simulink model "AMPC_sCon"  (R2019b)
settings: Solver=FixedStepAuto  StartTime=0.0  StopTime=Time(end)  FixedStep=0.025  RelTol=1e-3
libraries: neural x47, mpclib x1, cstblocks x1
(part 2 of 2)

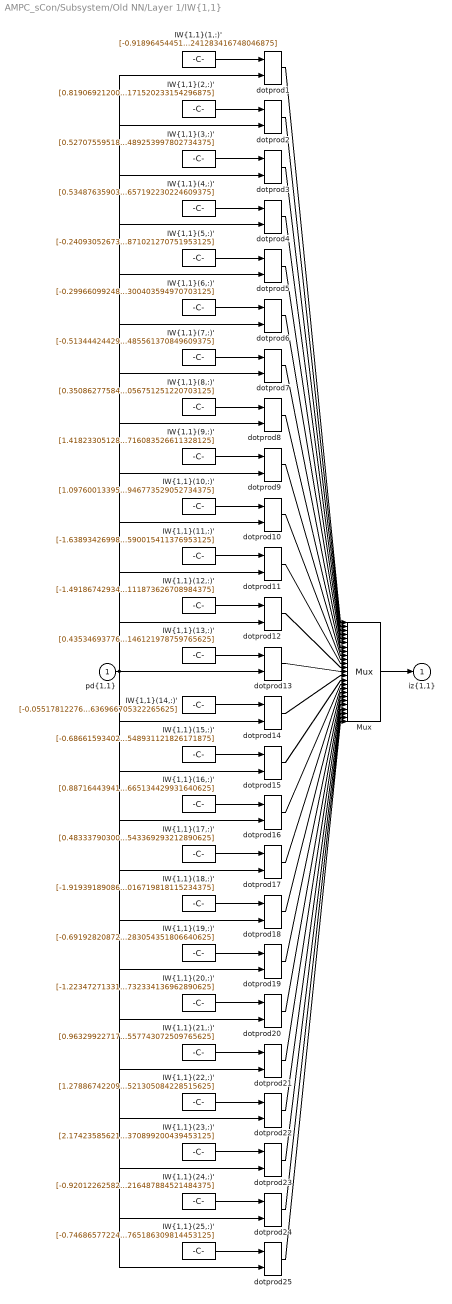
== system AMPC_sCon/Subsystem/Old NN/Layer 1/IW{1,1} ==
  "pd{1,1}" : Inport  PortDimensions=6
      mask Display: e = 0.06;c1 = [120 230 180]/255;c2 = ([120 230 180]+0)/(256+128);c3 = ([120 230 180]+128)/(256+128);patch([0 1 1 0],[0 0 1 1],c1);patch([0 1 1 1-e 1-e 0+e],[0 0 1 1-e 0+e 0+e],c2);patch([0 0 1 1-e 0+e 0+e],[0 1 1 1-e 1-e 0+e],c3);plot([0 1 1 0 0],[0 0 1 1 0]);
  "IW{1,1}(1,:)'" : Constant  Value=[-0.91896454451869669100005921791307628154754638671875;2.807406064374065923772150199511088430881500244140625;-0.32650530029088009609239406927372328937053680419921875;-0.68212399974366133559300351407728157937526702880859375;0.55443567787012237868538022667053155601024627685546875;-0.328157572076140435779478821132215671241283416748046875]
      mask Display: e = 0.06;c1 = [120 150 230]/255;c2 = ([120 150 230]+0)/383;c3 = ([120 150 230]+128)/383;patch([0 1 1 0],[0 0 1 1],c1);patch([0 1 1 1-e 1-e 0+e],[0 0 1 1-e 0+e 0+e],c2);patch([0 0 1 1-e 0+e 0+e],[0 1 1 1-e 1-e 0+e],c3);plot([0 1 1 0 0],[0 0 1 1 0]);disp('Weights');
  "IW{1,1}(10,:)'" : Constant  Value=[1.097600133959441226494391230517067015171051025390625;-0.07827061444567622039425458524419809691607952117919921875;-0.38990454765808413295502532491809688508510589599609375;0.46998928551050112023546034833998419344425201416015625;0.4354289920842753236485123125021345913410186767578125;-0.59819487501920798333543416447355411946773529052734375]
      mask Display: e = 0.06;c1 = [120 150 230]/255;c2 = ([120 150 230]+0)/383;c3 = ([120 150 230]+128)/383;patch([0 1 1 0],[0 0 1 1],c1);patch([0 1 1 1-e 1-e 0+e],[0 0 1 1-e 0+e 0+e],c2);patch([0 0 1 1-e 0+e 0+e],[0 1 1 1-e 1-e 0+e],c3);plot([0 1 1 0 0],[0 0 1 1 0]);disp('Weights');
  "IW{1,1}(11,:)'" : Constant  Value=[-1.6389342699858098217902124815736897289752960205078125;-0.7309100789032456635396783894975669682025909423828125;0.0018010659112654837758771275701974445837549865245819091796875;0.83129641458116487751084378032828681170940399169921875;-0.93893409236719238553092736765393055975437164306640625;0.084419703238978460735353337440756149590015411376953125]
      mask Display: e = 0.06;c1 = [120 150 230]/255;c2 = ([120 150 230]+0)/383;c3 = ([120 150 230]+128)/383;patch([0 1 1 0],[0 0 1 1],c1);patch([0 1 1 1-e 1-e 0+e],[0 0 1 1-e 0+e 0+e],c2);patch([0 0 1 1-e 0+e 0+e],[0 1 1 1-e 1-e 0+e],c3);plot([0 1 1 0 0],[0 0 1 1 0]);disp('Weights');
  "IW{1,1}(12,:)'" : Constant  Value=[-1.4918674293447633516507266904227435588836669921875;0.52049473620865904788246325551881454885005950927734375;-0.272842583889991330270419211956323124468326568603515625;-0.5921939615822207070294780351105146110057830810546875;-1.6000734146301442972770701089757494628429412841796875;-0.7163345210483613723084772573201917111873626708984375]
      mask Display: e = 0.06;c1 = [120 150 230]/255;c2 = ([120 150 230]+0)/383;c3 = ([120 150 230]+128)/383;patch([0 1 1 0],[0 0 1 1],c1);patch([0 1 1 1-e 1-e 0+e],[0 0 1 1-e 0+e 0+e],c2);patch([0 0 1 1-e 0+e 0+e],[0 1 1 1-e 1-e 0+e],c3);plot([0 1 1 0 0],[0 0 1 1 0]);disp('Weights');
  "IW{1,1}(13,:)'" : Constant  Value=[0.4353469377680905250116438764962367713451385498046875;-0.84085297783017975969954704851261340081691741943359375;-0.3262431999570882812378158632782287895679473876953125;-0.03343748267568195930987684505453216843307018280029296875;0.7569219535729778680632762188906781375408172607421875;-0.336770011411867520312313217800692655146121978759765625]
      mask Display: e = 0.06;c1 = [120 150 230]/255;c2 = ([120 150 230]+0)/383;c3 = ([120 150 230]+128)/383;patch([0 1 1 0],[0 0 1 1],c1);patch([0 1 1 1-e 1-e 0+e],[0 0 1 1-e 0+e 0+e],c2);patch([0 0 1 1-e 0+e 0+e],[0 1 1 1-e 1-e 0+e],c3);plot([0 1 1 0 0],[0 0 1 1 0]);disp('Weights');
  "IW{1,1}(14,:)'" : Constant  Value=[-0.055178122760997337648003480126135400496423244476318359375;-1.4381626335296340268854464738979004323482513427734375;0.1875648565884424356919879528504679910838603973388671875;-0.53640519002087516664545319144963286817073822021484375;-1.0068525371299339443709186525666154921054840087890625;0.160847593541183275789308027015067636966705322265625]
      mask Display: e = 0.06;c1 = [120 150 230]/255;c2 = ([120 150 230]+0)/383;c3 = ([120 150 230]+128)/383;patch([0 1 1 0],[0 0 1 1],c1);patch([0 1 1 1-e 1-e 0+e],[0 0 1 1-e 0+e 0+e],c2);patch([0 0 1 1-e 0+e 0+e],[0 1 1 1-e 1-e 0+e],c3);plot([0 1 1 0 0],[0 0 1 1 0]);disp('Weights');
  "IW{1,1}(15,:)'" : Constant  Value=[-0.686615934023023566368237879942171275615692138671875;0.426894044409089457037254078386467881500720977783203125;-0.60810228251544184985277752275578677654266357421875;0.1522748062778661870542151746121817268431186676025390625;-2.1099858845401460172297447570599615573883056640625;0.1713882654697056195924886878856341354548931121826171875]
      mask Display: e = 0.06;c1 = [120 150 230]/255;c2 = ([120 150 230]+0)/383;c3 = ([120 150 230]+128)/383;patch([0 1 1 0],[0 0 1 1],c1);patch([0 1 1 1-e 1-e 0+e],[0 0 1 1-e 0+e 0+e],c2);patch([0 0 1 1-e 0+e 0+e],[0 1 1 1-e 1-e 0+e],c3);plot([0 1 1 0 0],[0 0 1 1 0]);disp('Weights');
  "IW{1,1}(16,:)'" : Constant  Value=[0.88716443941147471452524086998892016708850860595703125;0.40313159970102241391742836640332825481891632080078125;-0.015657524645655340744809791431180201470851898193359375;-0.478263451738349443242981351431808434426784515380859375;0.3859891211729997717583273697528056800365447998046875;0.6315189817233604063773100278922356665134429931640625]
      mask Display: e = 0.06;c1 = [120 150 230]/255;c2 = ([120 150 230]+0)/383;c3 = ([120 150 230]+128)/383;patch([0 1 1 0],[0 0 1 1],c1);patch([0 1 1 1-e 1-e 0+e],[0 0 1 1-e 0+e 0+e],c2);patch([0 0 1 1-e 0+e 0+e],[0 1 1 1-e 1-e 0+e],c3);plot([0 1 1 0 0],[0 0 1 1 0]);disp('Weights');
  "IW{1,1}(17,:)'" : Constant  Value=[0.48333790300379242399486656722729094326496124267578125;0.0251588125096972210770207567520628799684345722198486328125;-0.67153040371300332100901187004637904465198516845703125;0.46244925298389250034603037420311011373996734619140625;-0.126361383991284270678079337812960147857666015625;-0.9536652713805617853637386360787786543369293212890625]
      mask Display: e = 0.06;c1 = [120 150 230]/255;c2 = ([120 150 230]+0)/383;c3 = ([120 150 230]+128)/383;patch([0 1 1 0],[0 0 1 1],c1);patch([0 1 1 1-e 1-e 0+e],[0 0 1 1-e 0+e 0+e],c2);patch([0 0 1 1-e 0+e 0+e],[0 1 1 1-e 1-e 0+e],c3);plot([0 1 1 0 0],[0 0 1 1 0]);disp('Weights');
  "IW{1,1}(18,:)'" : Constant  Value=[-1.919391890863494598562510873307473957538604736328125;2.760761832853932506992578055360354483127593994140625;0.166517652488541612054717688806704245507717132568359375;0.554430338119628718374087839038111269474029541015625;0.9634316882260487435729601202183403074741363525390625;-1.5238850536123587087189434896572493016719818115234375]
      mask Display: e = 0.06;c1 = [120 150 230]/255;c2 = ([120 150 230]+0)/383;c3 = ([120 150 230]+128)/383;patch([0 1 1 0],[0 0 1 1],c1);patch([0 1 1 1-e 1-e 0+e],[0 0 1 1-e 0+e 0+e],c2);patch([0 0 1 1-e 0+e 0+e],[0 1 1 1-e 1-e 0+e],c3);plot([0 1 1 0 0],[0 0 1 1 0]);disp('Weights');
  "IW{1,1}(19,:)'" : Constant  Value=[-0.69192820872236715512570981445605866611003875732421875;-1.0115896887588913255484612818690948188304901123046875;0.2082050329143752265270705947841634042561054229736328125;1.4276170938064451920723740840912796556949615478515625;0.60289644057316038594507290326873771846294403076171875;0.491245567452074427539088219418772496283054351806640625]
      mask Display: e = 0.06;c1 = [120 150 230]/255;c2 = ([120 150 230]+0)/383;c3 = ([120 150 230]+128)/383;patch([0 1 1 0],[0 0 1 1],c1);patch([0 1 1 1-e 1-e 0+e],[0 0 1 1-e 0+e 0+e],c2);patch([0 0 1 1-e 0+e 0+e],[0 1 1 1-e 1-e 0+e],c3);plot([0 1 1 0 0],[0 0 1 1 0]);disp('Weights');
  "IW{1,1}(2,:)'" : Constant  Value=[0.819069212007324409796638065017759799957275390625;1.4205841344905445478019601068808697164058685302734375;-0.2087539526108411480631588119649677537381649017333984375;0.5615055630163883204630792533862404525279998779296875;0.7621159660466625407337915021344088017940521240234375;-0.25482421381122211112568720636772923171520233154296875]
      mask Display: e = 0.06;c1 = [120 150 230]/255;c2 = ([120 150 230]+0)/383;c3 = ([120 150 230]+128)/383;patch([0 1 1 0],[0 0 1 1],c1);patch([0 1 1 1-e 1-e 0+e],[0 0 1 1-e 0+e 0+e],c2);patch([0 0 1 1-e 0+e 0+e],[0 1 1 1-e 1-e 0+e],c3);plot([0 1 1 0 0],[0 0 1 1 0]);disp('Weights');
  "IW{1,1}(20,:)'" : Constant  Value=[-1.223472713315403748168819220154546201229095458984375;1.02781452349469848428498153225518763065338134765625;-0.5016143513805861875454183973488397896289825439453125;-0.76512208370276379998387028535944409668445587158203125;-0.343872743653884926917640996180125512182712554931640625;-0.8302771328935032446594277644180692732334136962890625]
      mask Display: e = 0.06;c1 = [120 150 230]/255;c2 = ([120 150 230]+0)/383;c3 = ([120 150 230]+128)/383;patch([0 1 1 0],[0 0 1 1],c1);patch([0 1 1 1-e 1-e 0+e],[0 0 1 1-e 0+e 0+e],c2);patch([0 0 1 1-e 0+e 0+e],[0 1 1 1-e 1-e 0+e],c3);plot([0 1 1 0 0],[0 0 1 1 0]);disp('Weights');
  "IW{1,1}(21,:)'" : Constant  Value=[0.96329922717340188409451684492523781955242156982421875;-0.6551169661280218381449458320275880396366119384765625;-0.50582440032005393515390778702567331492900848388671875;0.046064824593341609226815336342042428441345691680908203125;1.406097969527585700433292004163376986980438232421875;-1.30481552967731406766915824846364557743072509765625]
      mask Display: e = 0.06;c1 = [120 150 230]/255;c2 = ([120 150 230]+0)/383;c3 = ([120 150 230]+128)/383;patch([0 1 1 0],[0 0 1 1],c1);patch([0 1 1 1-e 1-e 0+e],[0 0 1 1-e 0+e 0+e],c2);patch([0 0 1 1-e 0+e 0+e],[0 1 1 1-e 1-e 0+e],c3);plot([0 1 1 0 0],[0 0 1 1 0]);disp('Weights');
  "IW{1,1}(22,:)'" : Constant  Value=[1.2788674220914140189364616162492893636226654052734375;-0.499205108866402846867771359029575251042842864990234375;0.12542267272189933091652846997021697461605072021484375;-0.54779174719712830921025670249946415424346923828125;0.97010399881503683872097099083475768566131591796875;0.613862465609015917067381451488472521305084228515625]
      mask Display: e = 0.06;c1 = [120 150 230]/255;c2 = ([120 150 230]+0)/383;c3 = ([120 150 230]+128)/383;patch([0 1 1 0],[0 0 1 1],c1);patch([0 1 1 1-e 1-e 0+e],[0 0 1 1-e 0+e 0+e],c2);patch([0 0 1 1-e 0+e 0+e],[0 1 1 1-e 1-e 0+e],c3);plot([0 1 1 0 0],[0 0 1 1 0]);disp('Weights');
  "IW{1,1}(23,:)'" : Constant  Value=[2.1742358562138814903619277174584567546844482421875;0.7779663865511003972841308495844714343547821044921875;0.11376764528600201431540739349657087586820125579833984375;-0.321381834602109339726894177147187292575836181640625;0.31338586648281763213930162237375043332576751708984375;0.8184780163425291465983946181950159370899200439453125]
      mask Display: e = 0.06;c1 = [120 150 230]/255;c2 = ([120 150 230]+0)/383;c3 = ([120 150 230]+128)/383;patch([0 1 1 0],[0 0 1 1],c1);patch([0 1 1 1-e 1-e 0+e],[0 0 1 1-e 0+e 0+e],c2);patch([0 0 1 1-e 0+e 0+e],[0 1 1 1-e 1-e 0+e],c3);plot([0 1 1 0 0],[0 0 1 1 0]);disp('Weights');
  "IW{1,1}(24,:)'" : Constant  Value=[-0.920122625825073203742476835031993687152862548828125;1.7985903786357282374552823966951109468936920166015625;-0.449335796921472019338494874318712390959262847900390625;0.37211945524182443723049118489143438637256622314453125;-0.268179811625878616876406113078701309859752655029296875;-0.99187628535014782382717157815932296216487884521484375]
      mask Display: e = 0.06;c1 = [120 150 230]/255;c2 = ([120 150 230]+0)/383;c3 = ([120 150 230]+128)/383;patch([0 1 1 0],[0 0 1 1],c1);patch([0 1 1 1-e 1-e 0+e],[0 0 1 1-e 0+e 0+e],c2);patch([0 0 1 1-e 0+e 0+e],[0 1 1 1-e 1-e 0+e],c3);plot([0 1 1 0 0],[0 0 1 1 0]);disp('Weights');
  "IW{1,1}(25,:)'" : Constant  Value=[-0.7468657722437128665404770799796096980571746826171875;0.9514243031970905928318416044930927455425262451171875;-0.19912347847005718026736076353699900209903717041015625;0.42273079982580286095839028348564170300960540771484375;-0.454298439023558542348979472080827690660953521728515625;0.1158651407635991337219394381463644094765186309814453125]
      mask Display: e = 0.06;c1 = [120 150 230]/255;c2 = ([120 150 230]+0)/383;c3 = ([120 150 230]+128)/383;patch([0 1 1 0],[0 0 1 1],c1);patch([0 1 1 1-e 1-e 0+e],[0 0 1 1-e 0+e 0+e],c2);patch([0 0 1 1-e 0+e 0+e],[0 1 1 1-e 1-e 0+e],c3);plot([0 1 1 0 0],[0 0 1 1 0]);disp('Weights');
  "IW{1,1}(3,:)'" : Constant  Value=[0.52707559518076940729969237509067170321941375732421875;-1.35807461272378393601911739096976816654205322265625;0.6803855694700444711742193248937837779521942138671875;0.5457109471856937954470367913017980754375457763671875;-0.87266721000643909800231767803779803216457366943359375;0.354606028999767397547060454598977230489253997802734375]
      mask Display: e = 0.06;c1 = [120 150 230]/255;c2 = ([120 150 230]+0)/383;c3 = ([120 150 230]+128)/383;patch([0 1 1 0],[0 0 1 1],c1);patch([0 1 1 1-e 1-e 0+e],[0 0 1 1-e 0+e 0+e],c2);patch([0 0 1 1-e 0+e 0+e],[0 1 1 1-e 1-e 0+e],c3);plot([0 1 1 0 0],[0 0 1 1 0]);disp('Weights');
  "IW{1,1}(4,:)'" : Constant  Value=[0.5348763590344882690175154493772424757480621337890625;-2.94460120006832237748994884896092116832733154296875;0.25881394439468252688385518922586925327777862548828125;-0.988869737367270573713540215976536273956298828125;-1.34291304141692702245336477062664926052093505859375;0.8873294643855762497963723944849334657192230224609375]
      mask Display: e = 0.06;c1 = [120 150 230]/255;c2 = ([120 150 230]+0)/383;c3 = ([120 150 230]+128)/383;patch([0 1 1 0],[0 0 1 1],c1);patch([0 1 1 1-e 1-e 0+e],[0 0 1 1-e 0+e 0+e],c2);patch([0 0 1 1-e 0+e 0+e],[0 1 1 1-e 1-e 0+e],c3);plot([0 1 1 0 0],[0 0 1 1 0]);disp('Weights');
  "IW{1,1}(5,:)'" : Constant  Value=[-0.2409305267371661951614214558503590524196624755859375;1.3517602448933578873635497075156308710575103759765625;0.671714233157041373800666406168602406978607177734375;0.1699364545961201400370299552378128282725811004638671875;1.4733154643789483362326109272544272243976593017578125;0.44108263254802881903060551849193871021270751953125]
      mask Display: e = 0.06;c1 = [120 150 230]/255;c2 = ([120 150 230]+0)/383;c3 = ([120 150 230]+128)/383;patch([0 1 1 0],[0 0 1 1],c1);patch([0 1 1 1-e 1-e 0+e],[0 0 1 1-e 0+e 0+e],c2);patch([0 0 1 1-e 0+e 0+e],[0 1 1 1-e 1-e 0+e],c3);plot([0 1 1 0 0],[0 0 1 1 0]);disp('Weights');
  "IW{1,1}(6,:)'" : Constant  Value=[-0.29966099248417654710152646657661534845829010009765625;2.155080979873955637771132387570105493068695068359375;-0.5456468341177356240478957261075265705585479736328125;1.29078953244448957349277407047338783740997314453125;0.66091237151677351135958815575577318668365478515625;0.7268233797996483946946000287425704300403594970703125]
      mask Display: e = 0.06;c1 = [120 150 230]/255;c2 = ([120 150 230]+0)/383;c3 = ([120 150 230]+128)/383;patch([0 1 1 0],[0 0 1 1],c1);patch([0 1 1 1-e 1-e 0+e],[0 0 1 1-e 0+e 0+e],c2);patch([0 0 1 1-e 0+e 0+e],[0 1 1 1-e 1-e 0+e],c3);plot([0 1 1 0 0],[0 0 1 1 0]);disp('Weights');
  "IW{1,1}(7,:)'" : Constant  Value=[-0.5134442442948008444858487564488314092159271240234375;-0.046290477876960854641819054222651175223290920257568359375;-0.2734432707170408871633071612450294196605682373046875;-0.2045817861686594352210732949970406480133533477783203125;0.6178838573936122902097167752799578011035919189453125;0.8082262562382600545873856390244327485561370849609375]
      mask Display: e = 0.06;c1 = [120 150 230]/255;c2 = ([120 150 230]+0)/383;c3 = ([120 150 230]+128)/383;patch([0 1 1 0],[0 0 1 1],c1);patch([0 1 1 1-e 1-e 0+e],[0 0 1 1-e 0+e 0+e],c2);patch([0 0 1 1-e 0+e 0+e],[0 1 1 1-e 1-e 0+e],c3);plot([0 1 1 0 0],[0 0 1 1 0]);disp('Weights');
  "IW{1,1}(8,:)'" : Constant  Value=[0.350862775841264851184320150423445738852024078369140625;0.68910283718495712879104075909708626568317413330078125;0.401025938922157598742757045329199172556400299072265625;0.0211565590218434108893408307494610198773443698883056640625;-1.279037208798537772480585772427730262279510498046875;1.401791982737751851573193562217056751251220703125]
      mask Display: e = 0.06;c1 = [120 150 230]/255;c2 = ([120 150 230]+0)/383;c3 = ([120 150 230]+128)/383;patch([0 1 1 0],[0 0 1 1],c1);patch([0 1 1 1-e 1-e 0+e],[0 0 1 1-e 0+e 0+e],c2);patch([0 0 1 1-e 0+e 0+e],[0 1 1 1-e 1-e 0+e],c3);plot([0 1 1 0 0],[0 0 1 1 0]);disp('Weights');
  "IW{1,1}(9,:)'" : Constant  Value=[1.418233051281720946690256823785603046417236328125;-1.182436857788876860553273218101821839809417724609375;-0.96678645577470512240125799507950432598590850830078125;-0.1518551314846387223500556729050003923475742340087890625;-0.86831624417003328009201368331559933722019195556640625;-0.64704123302700822240041134136845357716083526611328125]
      mask Display: e = 0.06;c1 = [120 150 230]/255;c2 = ([120 150 230]+0)/383;c3 = ([120 150 230]+128)/383;patch([0 1 1 0],[0 0 1 1],c1);patch([0 1 1 1-e 1-e 0+e],[0 0 1 1-e 0+e 0+e],c2);patch([0 0 1 1-e 0+e 0+e],[0 1 1 1-e 1-e 0+e],c3);plot([0 1 1 0 0],[0 0 1 1 0]);disp('Weights');
  Mux : Mux  Inputs=25
      mask Display: e = 0.06;c1 = [120 150 230]/255;c2 = ([120 150 230]+0)/383;c3 = ([120 150 230]+128)/383;patch([0 1 1 0],[0 0 1 1],c1);patch([0 1 1 1-e 1-e 0+e],[0 0 1 1-e 0+e 0+e],c2);patch([0 0 1 1-e 0+e 0+e],[0 1 1 1-e 1-e 0+e],c3);plot([0 1 1 0 0],[0 0 1 1 0]);disp('Mux');
  dotprod{1..25} (25 alike) : neural/Weight Functions/dotprod
      settings: SourceProductName=MATLAB Runtime - Deep Learning Toolbox  SourceProductBaseCode=Missing
  "iz{1,1}" : Outport  VectorParamsAs1DForOutWhenUnconnected=off
      mask Display: e = 0.06;c1 = [120 230 180]/255;c2 = ([120 230 180]+0)/(256+128);c3 = ([120 230 180]+128)/(256+128);patch([0 1 1 0],[0 0 1 1],c1);patch([0 1 1 1-e 1-e 0+e],[0 0 1 1-e 0+e 0+e],c2);patch([0 0 1 1-e 0+e 0+e],[0 1 1 1-e 1-e 0+e],c3);plot([0 1 1 0 0],[0 0 1 1 0]);
  wires:
  "IW{1,1}(1,:)'"/1 -> dotprod1/1
  "pd{1,1}"/1 -> dotprod1/2, dotprod2/2, dotprod3/2, dotprod4/2, dotprod5/2, dotprod6/2, dotprod7/2, dotprod8/2, dotprod9/2, dotprod10/2, dotprod11/2, dotprod12/2, dotprod13/2, dotprod14/2, dotprod15/2, dotprod16/2, dotprod17/2, dotprod18/2, dotprod19/2, dotprod20/2, dotprod21/2, dotprod22/2, dotprod23/2, dotprod24/2, dotprod25/2
  dotprod1/1 -> Mux/1
  "IW{1,1}(2,:)'"/1 -> dotprod2/1
  dotprod2/1 -> Mux/2
  "IW{1,1}(3,:)'"/1 -> dotprod3/1
  dotprod3/1 -> Mux/3
  "IW{1,1}(4,:)'"/1 -> dotprod4/1
  dotprod4/1 -> Mux/4
  "IW{1,1}(5,:)'"/1 -> dotprod5/1
  dotprod5/1 -> Mux/5
  "IW{1,1}(6,:)'"/1 -> dotprod6/1
  dotprod6/1 -> Mux/6
  "IW{1,1}(7,:)'"/1 -> dotprod7/1
  dotprod7/1 -> Mux/7
  "IW{1,1}(8,:)'"/1 -> dotprod8/1
  dotprod8/1 -> Mux/8
  "IW{1,1}(9,:)'"/1 -> dotprod9/1
  dotprod9/1 -> Mux/9
  "IW{1,1}(10,:)'"/1 -> dotprod10/1
  dotprod10/1 -> Mux/10
  "IW{1,1}(11,:)'"/1 -> dotprod11/1
  dotprod11/1 -> Mux/11
  "IW{1,1}(12,:)'"/1 -> dotprod12/1
  dotprod12/1 -> Mux/12
  "IW{1,1}(13,:)'"/1 -> dotprod13/1
  dotprod13/1 -> Mux/13
  "IW{1,1}(14,:)'"/1 -> dotprod14/1
  dotprod14/1 -> Mux/14
  "IW{1,1}(15,:)'"/1 -> dotprod15/1
  dotprod15/1 -> Mux/15
  "IW{1,1}(16,:)'"/1 -> dotprod16/1
  dotprod16/1 -> Mux/16
  "IW{1,1}(17,:)'"/1 -> dotprod17/1
  dotprod17/1 -> Mux/17
  "IW{1,1}(18,:)'"/1 -> dotprod18/1
  dotprod18/1 -> Mux/18
  "IW{1,1}(19,:)'"/1 -> dotprod19/1
  dotprod19/1 -> Mux/19
  "IW{1,1}(20,:)'"/1 -> dotprod20/1
  dotprod20/1 -> Mux/20
  "IW{1,1}(21,:)'"/1 -> dotprod21/1
  dotprod21/1 -> Mux/21
  "IW{1,1}(22,:)'"/1 -> dotprod22/1
  dotprod22/1 -> Mux/22
  "IW{1,1}(23,:)'"/1 -> dotprod23/1
  dotprod23/1 -> Mux/23
  "IW{1,1}(24,:)'"/1 -> dotprod24/1
  dotprod24/1 -> Mux/24
  "IW{1,1}(25,:)'"/1 -> dotprod25/1
  dotprod25/1 -> Mux/25
  Mux/1 -> "iz{1,1}"/1

== system AMPC_sCon/Subsystem/Old NN/Layer 2/Delays 1 ==
  "p{2}" : Inport  PortDimensions=25
      mask Display: e = 0.06;c1 = [120 230 180]/255;c2 = ([120 230 180]+0)/(256+128);c3 = ([120 230 180]+128)/(256+128);patch([0 1 1 0],[0 0 1 1],c1);patch([0 1 1 1-e 1-e 0+e],[0 0 1 1-e 0+e 0+e],c2);patch([0 0 1 1-e 0+e 0+e],[0 1 1 1-e 1-e 0+e],c3);plot([0 1 1 0 0],[0 0 1 1 0]);
  mux : Mux  Inputs=1
      mask Display: e = 0.06;c1 = [120 150 230]/255;c2 = ([120 150 230]+0)/383;c3 = ([120 150 230]+128)/383;patch([0 1 1 0],[0 0 1 1],c1);patch([0 1 1 1-e 1-e 0+e],[0 0 1 1-e 0+e 0+e],c2);patch([0 0 1 1-e 0+e 0+e],[0 1 1 1-e 1-e 0+e],c3);plot([0 1 1 0 0],[0 0 1 1 0]);disp('Mux')
  "pd{2,1}" : Outport  VectorParamsAs1DForOutWhenUnconnected=off
      mask Display: e = 0.06;c1 = [120 230 180]/255;c2 = ([120 230 180]+0)/(256+128);c3 = ([120 230 180]+128)/(256+128);patch([0 1 1 0],[0 0 1 1],c1);patch([0 1 1 1-e 1-e 0+e],[0 0 1 1-e 0+e 0+e],c2);patch([0 0 1 1-e 0+e 0+e],[0 1 1 1-e 1-e 0+e],c3);plot([0 1 1 0 0],[0 0 1 1 0]);
  wires:
  "p{2}"/1 -> mux/1
  mux/1 -> "pd{2,1}"/1

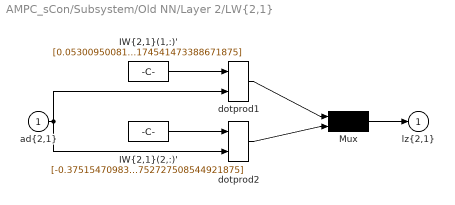
== system AMPC_sCon/Subsystem/Old NN/Layer 2/LW{2,1} ==
  "ad{2,1}" : Inport  PortDimensions=25
      mask Display: e = 0.06;c1 = [120 230 180]/255;c2 = ([120 230 180]+0)/(256+128);c3 = ([120 230 180]+128)/(256+128);patch([0 1 1 0],[0 0 1 1],c1);patch([0 1 1 1-e 1-e 0+e],[0 0 1 1-e 0+e 0+e],c2);patch([0 0 1 1-e 0+e 0+e],[0 1 1 1-e 1-e 0+e],c3);plot([0 1 1 0 0],[0 0 1 1 0]);
  "IW{2,1}(1,:)'" : Constant  Value=[0.053009500816631381636678810309604159556329250335693359375;1.068751779914871580245971927070058882236480712890625;0.8941755927975811868435584983672015368938446044921875;0.26666444265424960047283775566029362380504608154296875;1.9854215559896750686874611346866004168987274169921875;-0.061996390584446968430309965469859889708459377288818359375;-0.7599389840378567573253576483693905174732208251953125;-1.8953198972188689541695794105180539190769195556640625;1.27710150044223968990309003856964409351348876953125;1.0818234522679277542778208953677676618099212646484375;-1.9013012190243989696369908415363170206546783447265625;-1.4565290884924582126558334493893198668956756591796875;1.0871454996625884437122522285790182650089263916015625;1.18916750699715034755854503600858151912689208984375;-0.77329469543329254488384094656794331967830657958984375;-1.335247753105627932512788902386091649532318115234375;1.1370794018775078892957708376343362033367156982421875;0.292394494133218108000704660298652015626430511474609375;0.6910969489126503884079966155695728957653045654296875;1.5160004719763315872427256181254051625728607177734375;-1.3721078286370211873901325816405005753040313720703125;1.292941555738996495250603402382694184780120849609375;1.7138796645551959141329234626027755439281463623046875;-0.035139365064529477777899302282094140537083148956298828125;1.12598493238334196320238334010355174541473388671875]
      mask Display: e = 0.06;c1 = [120 150 230]/255;c2 = ([120 150 230]+0)/383;c3 = ([120 150 230]+128)/383;patch([0 1 1 0],[0 0 1 1],c1);patch([0 1 1 1-e 1-e 0+e],[0 0 1 1-e 0+e 0+e],c2);patch([0 0 1 1-e 0+e 0+e],[0 1 1 1-e 1-e 0+e],c3);plot([0 1 1 0 0],[0 0 1 1 0]);disp('weights');
  "IW{2,1}(2,:)'" : Constant  Value=[-0.3751547098353940068449219324975274503231048583984375;-0.91417283342699329207192704416229389607906341552734375;-0.17281979492504173645528453562292270362377166748046875;-1.107118138034655085988333667046390473842620849609375;0.1458148742536761466315198276788578368723392486572265625;0.8540653003652973751513854949735105037689208984375;0.2284368701578295690612918633632943965494632720947265625;0.1643582400806844756591118539290619082748889923095703125;-0.06650142004198549006144247641714173369109630584716796875;1.001777741426220558196291676722466945648193359375;-0.65315945190090285432660266451421193778514862060546875;-1.2713911175420176125072657669079490005970001220703125;1.3505144018127486216229726778692565858364105224609375;0.60722141728468159715959018285502679646015167236328125;-1.3227244308739709577338317103567533195018768310546875;1.0715503565368120764134118871879763901233673095703125;-0.53168100644631699491782228506053797900676727294921875;-0.96267136789897300719331951768253929913043975830078125;-0.29745905442390474515690357293351553380489349365234375;0.32415387176602428187521809377358295023441314697265625;0.496952388036444148156078881584107875823974609375;-0.0420948037311068834487315371006843633949756622314453125;0.99207643348153717877124790902598761022090911865234375;0.97866322498576197030928369713365100324153900146484375;0.86695627674721442712524321905220858752727508544921875]
      mask Display: e = 0.06;c1 = [120 150 230]/255;c2 = ([120 150 230]+0)/383;c3 = ([120 150 230]+128)/383;patch([0 1 1 0],[0 0 1 1],c1);patch([0 1 1 1-e 1-e 0+e],[0 0 1 1-e 0+e 0+e],c2);patch([0 0 1 1-e 0+e 0+e],[0 1 1 1-e 1-e 0+e],c3);plot([0 1 1 0 0],[0 0 1 1 0]);disp('weights');
  Mux : Mux  Inputs=2
      mask Display: e = 0.06;c1 = [120 150 230]/255;c2 = ([120 150 230]+0)/383;c3 = ([120 150 230]+128)/383;patch([0 1 1 0],[0 0 1 1],c1);patch([0 1 1 1-e 1-e 0+e],[0 0 1 1-e 0+e 0+e],c2);patch([0 0 1 1-e 0+e 0+e],[0 1 1 1-e 1-e 0+e],c3);plot([0 1 1 0 0],[0 0 1 1 0]);disp('Mux');
  dotprod1 : neural/Weight Functions/dotprod
      settings: SourceProductName=MATLAB Runtime - Deep Learning Toolbox  SourceProductBaseCode=Missing
  dotprod2 : neural/Weight Functions/dotprod
      settings: SourceProductName=MATLAB Runtime - Deep Learning Toolbox  SourceProductBaseCode=Missing
  "lz{2,1}" : Outport  VectorParamsAs1DForOutWhenUnconnected=off
      mask Display: e = 0.06;c1 = [120 230 180]/255;c2 = ([120 230 180]+0)/(256+128);c3 = ([120 230 180]+128)/(256+128);patch([0 1 1 0],[0 0 1 1],c1);patch([0 1 1 1-e 1-e 0+e],[0 0 1 1-e 0+e 0+e],c2);patch([0 0 1 1-e 0+e 0+e],[0 1 1 1-e 1-e 0+e],c3);plot([0 1 1 0 0],[0 0 1 1 0]);
  wires:
  "IW{2,1}(1,:)'"/1 -> dotprod1/1
  "ad{2,1}"/1 -> dotprod1/2, dotprod2/2
  dotprod1/1 -> Mux/1
  "IW{2,1}(2,:)'"/1 -> dotprod2/1
  dotprod2/1 -> Mux/2
  Mux/1 -> "lz{2,1}"/1

== matlab function AMPC_sCon/Plant ==
  data: Vx input; Ac output; Cf input; Cr input; Bc output; Cc output; Dc output
function [Ac, Bc, Cc, Dc]  = fcn(Vx,Cf,Cr)

% Model parameters
m = 1650;
Iz = 3234;
lf = 1.4;
lr = 1.65;
l = lf + lr;
% Continuous-time model
a11 = (-Cf-Cr)/(m*Vx);
a12 = -1 + ((Cr*lr - Cf*lf)/(m*Vx^2));
a13 = 0;
a14 = 0;

a21 = (Cr*lr - Cf*lf)/Iz;
a22 = (-Cf*lf^2-Cr*lr^2)/(Iz*Vx);
a23 = 0;
a24 = 0;

a31 = (Cf.^2 + Cf*Cr)/(m*Vx);
a32 = (1 - (Cr*lr - Cf*lf)/(m*Vx*2))*Cf;
a33 = -lf^2*Cf/(Vx*Iz);
a34 = lf*lr*Cf/(Vx*Iz);

a41 = (Cf*Cr + Cr^2)/(m*Vx);
a42 = (1 - ((Cr*lr - Cf*lf)/(m*Vx^2)))*Cr;
a43 = Cr*lf*lr/(Vx*Iz);
a44 = -Cr*lr^2/(Vx*Iz);

b11 = Cf/(m*Vx);
b12 = 0;

b21 = Cf*lf/Iz;
b22 = 0;

b31 = -Cf^2/(m*Vx);
b32 = Cf;

b41 = -Cf*Cr/(m*Vx);
b42 = 0;

Ac = [a11 a12 a13 a14;
      a21 a22 a23 a24;
      a31 a32 a33 a34;
      a41 a42 a43 a44];
Bc = [b11 b12;
      b21 b22;
      b31 b32;
      b41 b42];     % Steering Control
  
Cc = eye(4);
Dc = zeros(4,2);

== matlab function AMPC_sCon/MATLAB Function1 ==
  data: Vx input; A output size=[4,4]; Cf input; Cr input; steer input; x input size=[2,1]; B output size=[4,2]; C output size=[2,4]; D output size=[2,2]; U output size=[2,1]; Y output size=[4,1]; X output size=[2,1]; DX output size=[4,1]
function [A,B,C,D,U,Y,X,DX] = fcn(Vx,Cf,Cr,steer,x)
% Sample time
Ts = 0.025;

% Model parameters
m = 1650;
Iz = 3234;
lf = 1.4;
lr = 1.65;
l = lf + lr;
% Continuous-time model
a11 = (-Cf-Cr)/(m*Vx);
a12 = -1 + ((Cr*lr - Cf*lf)/(m*Vx^2));
a13 = 0;
a14 = 0;

a21 = (Cr*lr - Cf*lf)/Iz;
a22 = (-Cf*lf^2-Cr*lr^2)/(Iz*Vx);
a23 = 0;
a24 = 0;

a31 = (Cf.^2 + Cf*Cr)/(m*Vx);
a32 = (1 - (Cr*lr - Cf*lf)/(m*Vx*2))*Cf;
a33 = -lf^2*Cf/(Vx*Iz);
a34 = lf*lr*Cf/(Vx*Iz);

a41 = (Cf*Cr + Cr^2)/(m*Vx);
a42 = (1 - ((Cr*lr - Cf*lf)/(m*Vx^2)))*Cr;
a43 = Cr*lf*lr/(Vx*Iz);
a44 = -Cr*lr^2/(Vx*Iz);

b11 = Cf/(m*Vx);
b12 = 0;

b21 = Cf*lf/Iz;
b22 = 0;

b31 = -Cf^2/(m*Vx);
b32 = Cf;

b41 = -Cf*Cr/(m*Vx);
b42 = 0;

Ac = [a11 a12 a13 a14;
      a21 a22 a23 a24;
      a31 a32 a33 a34;
      a41 a42 a43 a44];
Bc = [b11 b12;
      b21 b22;
      b31 b32;
      b41 b42];     % Steering Control
  
Cc = [1 0 0 0; 0 1 0 0];
Dc = zeros(2,2);



% Generate discrete-time model
nx = size(Ac,1);
nu = size(Bc,2);
M = expm([[Ac Bc]*Ts; zeros(nu,nx+nu)]);
A = M(1:nx,1:nx);
B = M(1:nx,nx+1:nx+nu);
C = Cc;
D = Dc;

% Nominal conditions for discrete-time plant
X = x;
U = steer;
Y = C*x + D*steer;
DX = A*x+B*steer-x;
